simulink subsystem "quatquad_controller_sim"  (R2021b)
settings: Solver=VariableStepAuto  StartTime=0.0  StopTime=10.0  RelTol=1e-3
values from neighbouring files (symbols this model uses):
  K_d1 = K_d1_lqr    [quatquad_main.m]
  K_d2 = K_d2_lqr    [quatquad_main.m]
  K_e = K_e_lqr    [quatquad_main.m]
  K_f = K_f_lqr    [quatquad_main.m]
  linearization_method = 1    [quatquad_main.m]
  S_c = [zeros(9,1),eye(9)]    [quatquad_analysis.m]
  u_eq = [9.81;0;0;0]    [quatquad_main.m]
undefined symbols (not defined in the file or in its folder): K_alt_f, K_att_f, K_attr_f, T_e
libraries: simulink x3
settings Model: Creator=vifre  LastModifiedBy=vifre

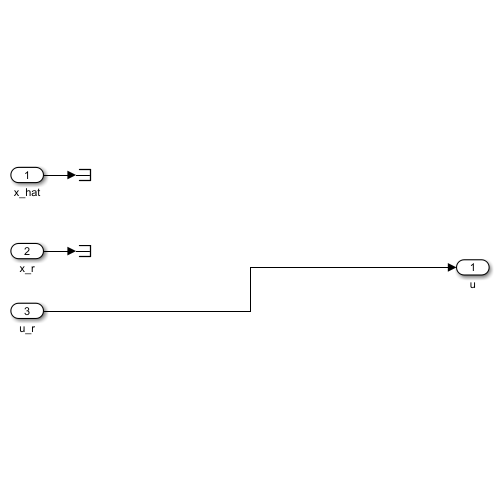
[thumbnail: Simulink's stored preview of the top-level diagram]
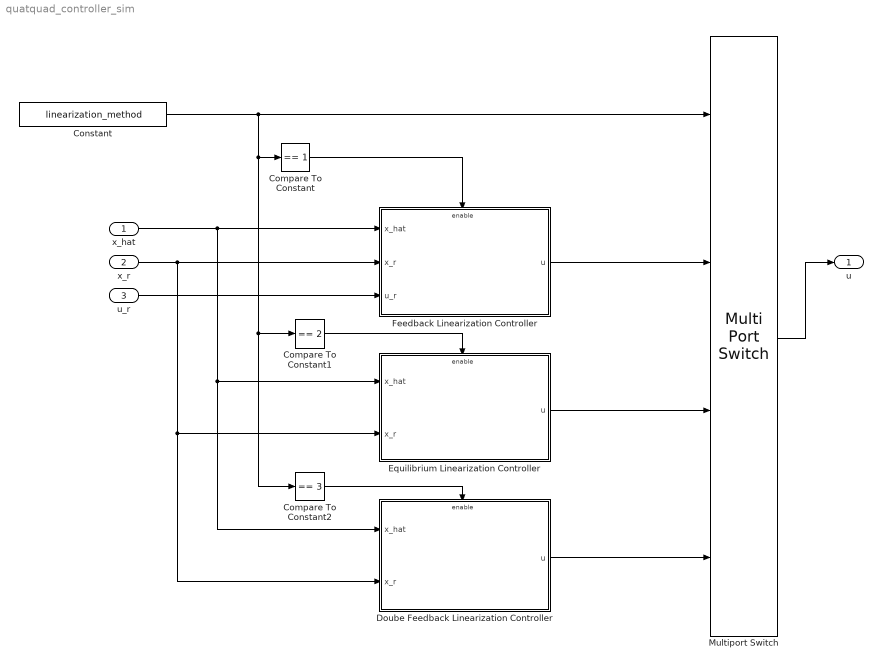
== system quatquad_controller_sim ==
  x_hat : Inport
  x_r : Inport  Port=2
  u_r : Inport  Port=3
  Compare To Constant : simulink/Logic and Bit Operations/Compare To Constant  relop===  const=1  OutDataTypeStr=boolean
  Compare To Constant1 : simulink/Logic and Bit Operations/Compare To Constant  relop===  const=2  OutDataTypeStr=boolean
  Compare To Constant2 : simulink/Logic and Bit Operations/Compare To Constant  relop===  const=3  OutDataTypeStr=boolean
  Constant : Constant  Value=linearization_method
  Doube Feedback Linearization Controller : Subsystem
  Equilibrium Linearization Controller : Subsystem
  Feedback Linearization Controller : Subsystem
  Multiport Switch : MultiPortSwitch
  u : Outport
  wires:
  x_hat/1 -> Doube Feedback Linearization Controller/1(x_hat), Equilibrium Linearization Controller/1(x_hat), Feedback Linearization Controller/1(x_hat)
  x_r/1 -> Doube Feedback Linearization Controller/2(x_r), Equilibrium Linearization Controller/2(x_r), Feedback Linearization Controller/2(x_r)
  u_r/1 -> Feedback Linearization Controller/3(u_r)
  Equilibrium Linearization Controller/1(u) -> Multiport Switch/3
  Multiport Switch/1 -> u/1
  Feedback Linearization Controller/1(u) -> Multiport Switch/2
  Constant/1 -> Compare To Constant/1, Compare To Constant1/1, Compare To Constant2/1, Multiport Switch/1
  Doube Feedback Linearization Controller/1(u) -> Multiport Switch/4
  Compare To Constant/1 -> Feedback Linearization Controller/Enable
  Compare To Constant1/1 -> Equilibrium Linearization Controller/Enable
  Compare To Constant2/1 -> Doube Feedback Linearization Controller/Enable

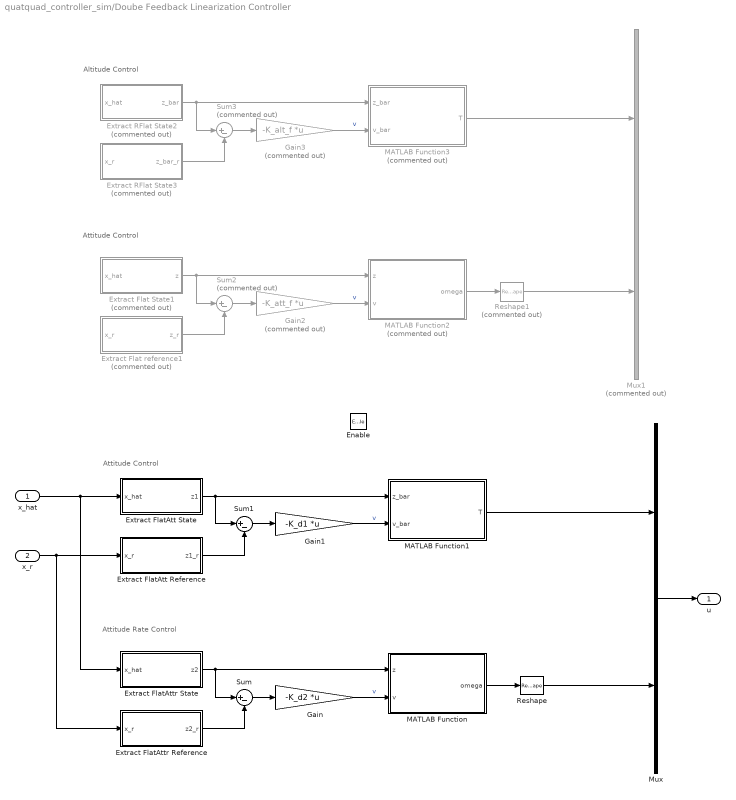
== system quatquad_controller_sim/Doube Feedback Linearization Controller ==
  note: Attitude Control
  note: Attitude Rate Control
  note: Attitude Control
  note: Altitude Control
  x_hat : Inport
  x_r : Inport  Port=2
  Enable : EnablePort
  Extract Flat State1 : Subsystem  Commented=on
  Extract Flat reference1 : Subsystem  Commented=on
  Extract FlatAtt Reference : Subsystem
  Extract FlatAtt State : Subsystem
  Extract FlatAttr Reference : Subsystem
  Extract FlatAttr State : Subsystem
  Extract RFlat State2 : Subsystem  Commented=on
  Extract RFlat State3 : Subsystem  Commented=on
  Gain : Gain  Gain=-K_d2  Multiplication=Matrix(K*u) (u vector)
  Gain1 : Gain  Gain=-K_d1  Multiplication=Matrix(K*u) (u vector)
  Gain2 : Gain  Commented=on  Gain=-K_att_f  Multiplication=Matrix(K*u) (u vector)
  Gain3 : Gain  Commented=on  Gain=-K_alt_f  Multiplication=Matrix(K*u) (u vector)
  MATLAB Function : MATLAB Function  TreatAsAtomicUnit=on
  MATLAB Function1 : MATLAB Function  TreatAsAtomicUnit=on
  MATLAB Function2 : MATLAB Function  Commented=on  TreatAsAtomicUnit=on
  MATLAB Function3 : MATLAB Function  Commented=on  TreatAsAtomicUnit=on
  Mux : Mux  Inputs=2
  Mux1 : Mux  Commented=on  Inputs=2
  Reshape : Reshape
  Reshape1 : Reshape  Commented=on
  Sum : Sum  Inputs=|+-
  Sum1 : Sum  Inputs=|+-
  Sum2 : Sum  Commented=on  Inputs=|+-
  Sum3 : Sum  Commented=on  Inputs=|+-
  u : Outport
  wires:
  x_r/1 -> Extract FlatAtt Reference/1(x_r), Extract FlatAttr Reference/1(x_r)
  x_hat/1 -> Extract FlatAtt State/1(x_hat), Extract FlatAttr State/1(x_hat)
  Mux/1 -> u/1
  Extract FlatAttr State/1(z2) -> Sum/1, MATLAB Function/1(z)
  Gain/1 -> MATLAB Function/2(v)  "v"
  MATLAB Function/1(omega) -> Reshape/1
  Extract FlatAttr Reference/1(z2_r) -> Sum/2
  Sum/1 -> Gain/1
  Sum1/1 -> Gain1/1
  Extract FlatAtt Reference/1(z1_r) -> Sum1/2
  Gain1/1 -> MATLAB Function1/2(v_bar)  "v"
  Extract FlatAtt State/1(z1) -> Sum1/1, MATLAB Function1/1(z_bar)
  Reshape/1 -> Mux/2
  MATLAB Function1/1(T) -> Mux/1
  Gain3/1 -> MATLAB Function3/2(v_bar)  "v"
  Sum3/1 -> Gain3/1
  Reshape1/1 -> Mux1/2
  MATLAB Function3/1(T) -> Mux1/1
  Extract Flat State1/1(z) -> Sum2/1, MATLAB Function2/1(z)
  Sum2/1 -> Gain2/1
  Extract Flat reference1/1(z_r) -> Sum2/2
  Extract RFlat State3/1(z_bar_r) -> Sum3/2
  Extract RFlat State2/1(z_bar) -> Sum3/1, MATLAB Function3/1(z_bar)
  MATLAB Function2/1(omega) -> Reshape1/1
  Gain2/1 -> MATLAB Function2/2(v)  "v"

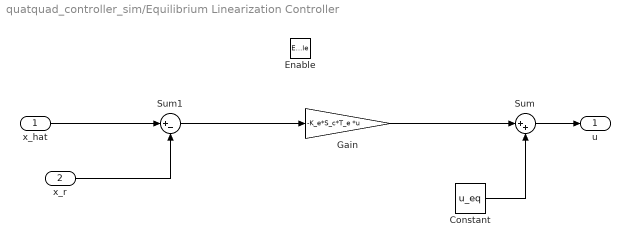
== system quatquad_controller_sim/Equilibrium Linearization Controller ==
  x_hat : Inport
  x_r : Inport  Port=2
  Enable : EnablePort
  Constant : Constant  Value=u_eq
  Gain : Gain  Gain=-K_e*S_c*T_e  Multiplication=Matrix(K*u) (u vector)
  Sum : Sum  Inputs=|++
  Sum1 : Sum  Inputs=|+-
  u : Outport
  wires:
  x_r/1 -> Sum1/2
  x_hat/1 -> Sum1/1
  Sum1/1 -> Gain/1
  Gain/1 -> Sum/1
  Constant/1 -> Sum/2
  Sum/1 -> u/1

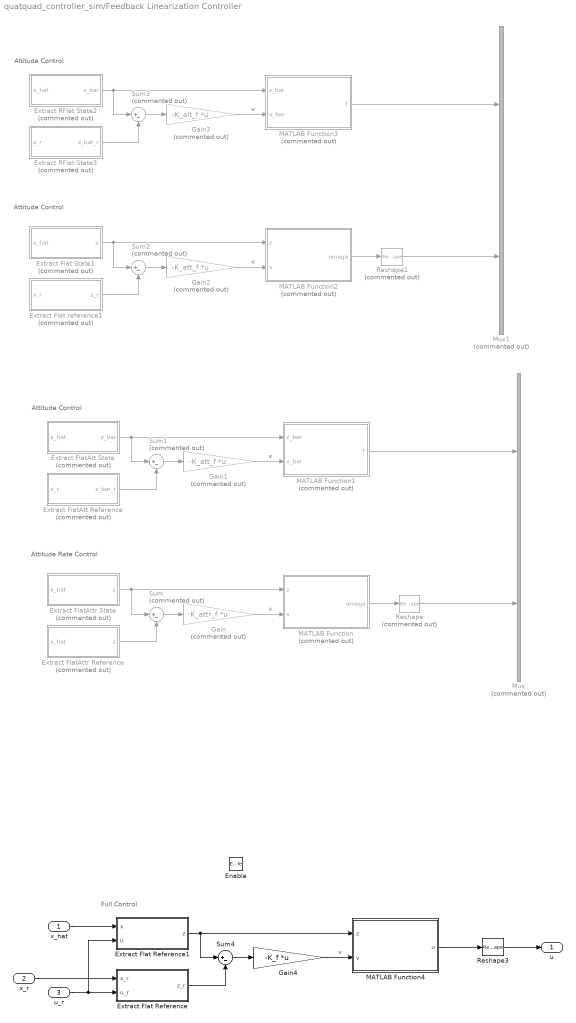
== system quatquad_controller_sim/Feedback Linearization Controller ==
  note: Full Control
  note: Altitude Control
  note: Attitude Control
  note: Attitude Rate Control
  note: Attitude Control
  x_hat : Inport
  x_r : Inport  Port=2
  u_r : Inport  Port=3
  Enable : EnablePort
  Extract Flat Reference : Subsystem
  Extract Flat Reference1 : Subsystem
  Extract Flat State1 : Subsystem  Commented=on
  Extract Flat reference1 : Subsystem  Commented=on
  Extract FlatAtt Reference : Subsystem  Commented=on
  Extract FlatAtt State : Subsystem  Commented=on
  Extract FlatAttr Reference : Subsystem  Commented=on
  Extract FlatAttr State : Subsystem  Commented=on
  Extract RFlat State2 : Subsystem  Commented=on
  Extract RFlat State3 : Subsystem  Commented=on
  Gain : Gain  Commented=on  Gain=-K_attr_f  Multiplication=Matrix(K*u) (u vector)
  Gain1 : Gain  Commented=on  Gain=-K_att_f  Multiplication=Matrix(K*u) (u vector)
  Gain2 : Gain  Commented=on  Gain=-K_att_f  Multiplication=Matrix(K*u) (u vector)
  Gain3 : Gain  Commented=on  Gain=-K_alt_f  Multiplication=Matrix(K*u) (u vector)
  Gain4 : Gain  Gain=-K_f  Multiplication=Matrix(K*u) (u vector)
  MATLAB Function : MATLAB Function  Commented=on  TreatAsAtomicUnit=on
  MATLAB Function1 : MATLAB Function  Commented=on  TreatAsAtomicUnit=on
  MATLAB Function2 : MATLAB Function  Commented=on  TreatAsAtomicUnit=on
  MATLAB Function3 : MATLAB Function  Commented=on  TreatAsAtomicUnit=on
  MATLAB Function4 : MATLAB Function  TreatAsAtomicUnit=on
  Mux : Mux  Commented=on  Inputs=2
  Mux1 : Mux  Commented=on  Inputs=2
  Reshape : Reshape  Commented=on
  Reshape1 : Reshape  Commented=on
  Reshape3 : Reshape
  Sum{,1..3} (4 alike) : Sum  Commented=on  Inputs=|+-
  Sum4 : Sum  Inputs=|+-
  u : Outport
  wires:
  u_r/1 -> Extract Flat Reference/2(u_r), Extract Flat Reference1/2(u)
  MATLAB Function4/1(u) -> Reshape3/1
  Extract Flat Reference1/1(z) -> MATLAB Function4/1(z), Sum4/1
  Extract Flat Reference/1(z_r) -> Sum4/2
  Gain4/1 -> MATLAB Function4/2(v)  "v"
  Sum4/1 -> Gain4/1
  x_r/1 -> Extract Flat Reference/1(x_r)
  x_hat/1 -> Extract Flat Reference1/1(x)
  Reshape3/1 -> u/1
  Gain2/1 -> MATLAB Function2/2(v)  "v"
  MATLAB Function2/1(omega) -> Reshape1/1
  Extract RFlat State2/1(z_bar) -> MATLAB Function3/1(z_bar), Sum3/1
  Extract RFlat State3/1(z_bar_r) -> Sum3/2
  Extract Flat reference1/1(z_r) -> Sum2/2
  Sum2/1 -> Gain2/1
  Extract Flat State1/1(z) -> MATLAB Function2/1(z), Sum2/1
  MATLAB Function3/1(T) -> Mux1/1
  Reshape1/1 -> Mux1/2
  Sum3/1 -> Gain3/1
  Gain3/1 -> MATLAB Function3/2(v_bar)  "v"
  MATLAB Function1/1(T) -> Mux/1
  Reshape/1 -> Mux/2
  Extract FlatAtt State/1(z_bar) -> MATLAB Function1/1(z_bar), Sum1/1
  Gain1/1 -> MATLAB Function1/2(v_bar)  "v"
  Extract FlatAtt Reference/1(z_bar_r) -> Sum1/2
  Sum1/1 -> Gain1/1
  Sum/1 -> Gain/1
  Extract FlatAttr Reference/1(z) -> Sum/2
  MATLAB Function/1(omega) -> Reshape/1
  Gain/1 -> MATLAB Function/2(v)  "v"
  Extract FlatAttr State/1(z) -> MATLAB Function/1(z), Sum/1

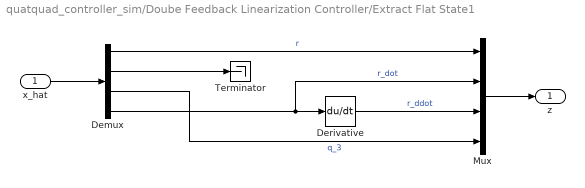
== system quatquad_controller_sim/Doube Feedback Linearization Controller/Extract Flat State1 ==
  x_hat : Inport
  Demux : Demux  Outputs=[3 3 1 3]
  Derivative : Derivative
  Mux : Mux
  Terminator : Terminator
  z : Outport
  wires:
  x_hat/1 -> Demux/1
  Demux/1 -> Mux/1  "r"
  Derivative/1 -> Mux/3  "r_ddot"
  Mux/1 -> z/1
  Demux/3 -> Mux/4  "q_3"
  Demux/2 -> Terminator/1
  Demux/4 -> Mux/2, Derivative/1  "r_dot"

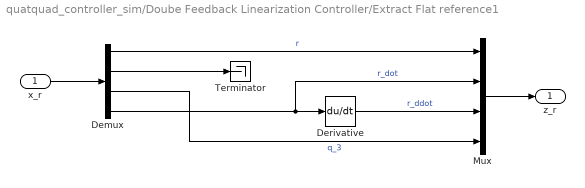
== system quatquad_controller_sim/Doube Feedback Linearization Controller/Extract Flat reference1 ==
  x_r : Inport
  Demux : Demux  Outputs=[3 3 1 3]
  Derivative : Derivative
  Mux : Mux
  Terminator : Terminator
  z_r : Outport
  wires:
  Demux/4 -> Derivative/1, Mux/2  "r_dot"
  Demux/2 -> Terminator/1
  Demux/3 -> Mux/4  "q_3"
  Mux/1 -> z_r/1
  Derivative/1 -> Mux/3  "r_ddot"
  Demux/1 -> Mux/1  "r"
  x_r/1 -> Demux/1

== system quatquad_controller_sim/Doube Feedback Linearization Controller/Extract FlatAtt Reference ==
  x_r : Inport
  Demux : Demux  Outputs=[3 4 3]
  Mux : Mux  Inputs=2
  Terminator : Terminator
  z1_r : Outport
  wires:
  Demux/3 -> Mux/2  "r_dot"
  x_r/1 -> Demux/1
  Demux/1 -> Mux/1  "r"
  Mux/1 -> z1_r/1
  Demux/2 -> Terminator/1

== system quatquad_controller_sim/Doube Feedback Linearization Controller/Extract FlatAtt State ==
  x_hat : Inport
  Demux : Demux  Outputs=[3 4 3]
  Mux : Mux  Inputs=2
  Terminator : Terminator
  z1 : Outport
  wires:
  Demux/2 -> Terminator/1
  Mux/1 -> z1/1
  Demux/1 -> Mux/1  "r"
  x_hat/1 -> Demux/1
  Demux/3 -> Mux/2  "r_dot"

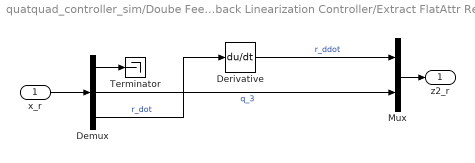
== system quatquad_controller_sim/Doube Feedback Linearization Controller/Extract FlatAttr Reference ==
  x_r : Inport
  Demux : Demux  Outputs=[6 1 3]
  Derivative : Derivative
  Mux : Mux  Inputs=2
  Terminator : Terminator
  z2_r : Outport
  wires:
  x_r/1 -> Demux/1
  Derivative/1 -> Mux/1  "r_ddot"
  Mux/1 -> z2_r/1
  Demux/1 -> Terminator/1
  Demux/2 -> Mux/2  "q_3"
  Demux/3 -> Derivative/1  "r_dot"

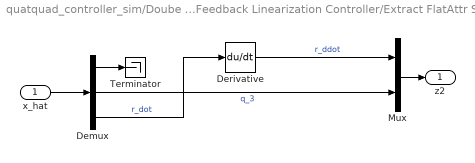
== system quatquad_controller_sim/Doube Feedback Linearization Controller/Extract FlatAttr State ==
  x_hat : Inport
  Demux : Demux  Outputs=[6 1 3]
  Derivative : Derivative
  Mux : Mux  Inputs=2
  Terminator : Terminator
  z2 : Outport
  wires:
  x_hat/1 -> Demux/1
  Derivative/1 -> Mux/1  "r_ddot"
  Mux/1 -> z2/1
  Demux/1 -> Terminator/1
  Demux/2 -> Mux/2  "q_3"
  Demux/3 -> Derivative/1  "r_dot"

== system quatquad_controller_sim/Doube Feedback Linearization Controller/Extract RFlat State2 ==
  x_hat : Inport
  Demux : Demux  Outputs=[3 4 3]
  Mux : Mux  Inputs=2
  Terminator : Terminator
  z_bar : Outport
  wires:
  Demux/2 -> Terminator/1
  Mux/1 -> z_bar/1
  Demux/1 -> Mux/1  "r"
  x_hat/1 -> Demux/1
  Demux/3 -> Mux/2  "r_dot"

== system quatquad_controller_sim/Doube Feedback Linearization Controller/Extract RFlat State3 ==
  x_r : Inport
  Demux : Demux  Outputs=[3 4 3]
  Mux : Mux  Inputs=2
  Terminator : Terminator
  z_bar_r : Outport
  wires:
  Demux/3 -> Mux/2  "r_dot"
  x_r/1 -> Demux/1
  Demux/1 -> Mux/1  "r"
  Mux/1 -> z_bar_r/1
  Demux/2 -> Terminator/1

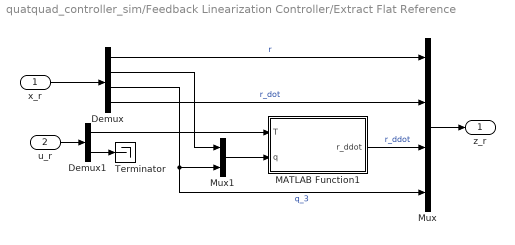
== system quatquad_controller_sim/Feedback Linearization Controller/Extract Flat Reference ==
  x_r : Inport
  u_r : Inport  Port=2
  Demux : Demux  Outputs=[3 3 1 3]
  Demux1 : Demux  Outputs=[1 3]
  MATLAB Function1 : MATLAB Function  TreatAsAtomicUnit=on
  Mux : Mux
  Mux1 : Mux  Inputs=2
  Terminator : Terminator
  z_r : Outport
  wires:
  u_r/1 -> Demux1/1
  Demux1/1 -> MATLAB Function1/1(T)
  Demux1/2 -> Terminator/1
  Mux1/1 -> MATLAB Function1/2(q)
  MATLAB Function1/1(r_ddot) -> Mux/3  "r_ddot"
  Demux/2 -> Mux1/1
  Mux/1 -> z_r/1
  Demux/1 -> Mux/1  "r"
  x_r/1 -> Demux/1
  Demux/4 -> Mux/2  "r_dot"
  Demux/3 -> Mux/4, Mux1/2  "q_3"

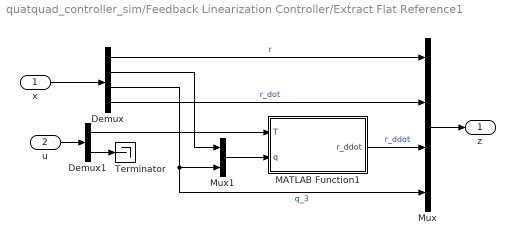
== system quatquad_controller_sim/Feedback Linearization Controller/Extract Flat Reference1 ==
  x : Inport
  u : Inport  Port=2
  Demux : Demux  Outputs=[3 3 1 3]
  Demux1 : Demux  Outputs=[1 3]
  MATLAB Function1 : MATLAB Function  TreatAsAtomicUnit=on
  Mux : Mux
  Mux1 : Mux  Inputs=2
  Terminator : Terminator
  z : Outport
  wires:
  Demux/3 -> Mux1/2, Mux/4  "q_3"
  Demux/4 -> Mux/2  "r_dot"
  x/1 -> Demux/1
  Demux/1 -> Mux/1  "r"
  Mux/1 -> z/1
  Demux/2 -> Mux1/1
  MATLAB Function1/1(r_ddot) -> Mux/3  "r_ddot"
  Mux1/1 -> MATLAB Function1/2(q)
  Demux1/2 -> Terminator/1
  Demux1/1 -> MATLAB Function1/1(T)
  u/1 -> Demux1/1

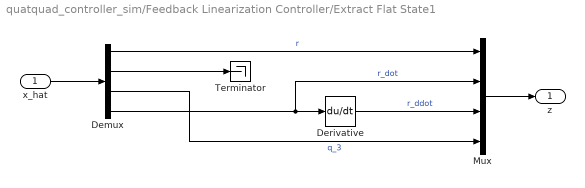
== system quatquad_controller_sim/Feedback Linearization Controller/Extract Flat State1 ==
  x_hat : Inport
  Demux : Demux  Outputs=[3 3 1 3]
  Derivative : Derivative
  Mux : Mux
  Terminator : Terminator
  z : Outport
  wires:
  Demux/4 -> Derivative/1, Mux/2  "r_dot"
  Demux/2 -> Terminator/1
  Demux/3 -> Mux/4  "q_3"
  Mux/1 -> z/1
  Derivative/1 -> Mux/3  "r_ddot"
  Demux/1 -> Mux/1  "r"
  x_hat/1 -> Demux/1

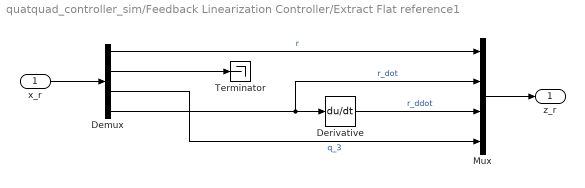
== system quatquad_controller_sim/Feedback Linearization Controller/Extract Flat reference1 ==
  x_r : Inport
  Demux : Demux  Outputs=[3 3 1 3]
  Derivative : Derivative
  Mux : Mux
  Terminator : Terminator
  z_r : Outport
  wires:
  x_r/1 -> Demux/1
  Demux/1 -> Mux/1  "r"
  Derivative/1 -> Mux/3  "r_ddot"
  Mux/1 -> z_r/1
  Demux/3 -> Mux/4  "q_3"
  Demux/2 -> Terminator/1
  Demux/4 -> Mux/2, Derivative/1  "r_dot"

== system quatquad_controller_sim/Feedback Linearization Controller/Extract FlatAtt Reference ==
  x_r : Inport
  Demux : Demux  Outputs=[3 4 3]
  Mux : Mux  Inputs=2
  Terminator : Terminator
  z_bar_r : Outport
  wires:
  Demux/2 -> Terminator/1
  Mux/1 -> z_bar_r/1
  Demux/1 -> Mux/1  "r"
  x_r/1 -> Demux/1
  Demux/3 -> Mux/2  "r_dot"

== system quatquad_controller_sim/Feedback Linearization Controller/Extract FlatAtt State ==
  x_hat : Inport
  Demux : Demux  Outputs=[3 4 3]
  Mux : Mux  Inputs=2
  Terminator : Terminator
  z_bar : Outport
  wires:
  Demux/3 -> Mux/2  "r_dot"
  x_hat/1 -> Demux/1
  Demux/1 -> Mux/1  "r"
  Mux/1 -> z_bar/1
  Demux/2 -> Terminator/1

== system quatquad_controller_sim/Feedback Linearization Controller/Extract FlatAttr Reference ==
  x_hat : Inport
  Demux : Demux  Outputs=[6 1 3]
  Derivative : Derivative
  Mux : Mux  Inputs=2
  Terminator : Terminator
  z : Outport
  wires:
  Demux/3 -> Derivative/1  "r_dot"
  Demux/2 -> Mux/2  "q_3"
  Demux/1 -> Terminator/1
  Mux/1 -> z/1
  Derivative/1 -> Mux/1  "r_ddot"
  x_hat/1 -> Demux/1

== system quatquad_controller_sim/Feedback Linearization Controller/Extract FlatAttr State ==
  x_hat : Inport
  Demux : Demux  Outputs=[6 1 3]
  Derivative : Derivative
  Mux : Mux  Inputs=2
  Terminator : Terminator
  z : Outport
  wires:
  Demux/3 -> Derivative/1  "r_dot"
  Demux/2 -> Mux/2  "q_3"
  Demux/1 -> Terminator/1
  Mux/1 -> z/1
  Derivative/1 -> Mux/1  "r_ddot"
  x_hat/1 -> Demux/1

== system quatquad_controller_sim/Feedback Linearization Controller/Extract RFlat State2 ==
  x_hat : Inport
  Demux : Demux  Outputs=[3 4 3]
  Mux : Mux  Inputs=2
  Terminator : Terminator
  z_bar : Outport
  wires:
  Demux/3 -> Mux/2  "r_dot"
  x_hat/1 -> Demux/1
  Demux/1 -> Mux/1  "r"
  Mux/1 -> z_bar/1
  Demux/2 -> Terminator/1

== system quatquad_controller_sim/Feedback Linearization Controller/Extract RFlat State3 ==
  x_r : Inport
  Demux : Demux  Outputs=[3 4 3]
  Mux : Mux  Inputs=2
  Terminator : Terminator
  z_bar_r : Outport
  wires:
  Demux/2 -> Terminator/1
  Mux/1 -> z_bar_r/1
  Demux/1 -> Mux/1  "r"
  x_r/1 -> Demux/1
  Demux/3 -> Mux/2  "r_dot"

== matlab function quatquad_controller_sim/Feedback Linearization Controller/MATLAB Function1 ==
  data: z_bar input; T output; v_bar input
function T = recover_att(z_bar, v_bar)
g = 9.81;
z_W = [0;0;1];
T = norm(v_bar + g*z_W);

== matlab function quatquad_controller_sim/Feedback Linearization Controller/MATLAB Function2 ==
  data: z input; omega output; v input
function omega = recover_att(z, v)
g = 9.81;
u = zeros(4,1);
r = z(1:3);
r_dot = z(4:6);
r_ddot = z(7:9);
q_3 = z(10);
r_dddot = v(1:3);
q_dot_3 = v(4);
z_W = [0;0;1];
T = norm(r_ddot+g*z_W);
q_0 = sqrt((r_ddot(3)+g)/T-q_3^2+1/2);
q_1 = (q_3*r_ddot(1) - q_0*r_ddot(2))/(2*T*(q_0^2+q_3^2));
q_2 = (q_0*r_ddot(1) + q_3*r_ddot(2))/(2*T*(q_0^2+q_3^2));
q = [q_0;q_1;q_2;q_3];
z_B = [2*(q(1)*q(3) + q(2)*q(4));
       -2*(q(1)*q(2) - q(3)*q(4));
       (q(1)^2 - q(2)^2 - q(3)^2 + q(4)^2)];
T_dot = dot(r_dddot,z_B);
q_dot_0 = 1/(2*q_0)*((T*r_dddot(3)-T_dot)/(2*T^2) - 2*q_3*q_dot_3);
num_q1 = q_3*r_ddot(1) - q_0*r_ddot(2);
num_q2 = q_0*r_ddot(1) + q_3*r_ddot(2);
num_q1_dot = q_dot_3*r_ddot(1) + q_3*r_dddot(1) - q_dot_0*r_ddot(2) - q_0*r_dddot(2);
num_q2_dot = q_dot_0*r_ddot(1) + q_0*r_dddot(1) + q_dot_3*r_ddot(2) + q_3*r_dddot(2); 
den = (2*T*(q_0^2 + q_3^2))^-1;
den_dot = -(2*T*(q_0^2+q_3^2))^(-2)*(2*T_dot*(q_0^2+q_3^2) + 2*T*(2*q_0*q_dot_0 + 2*q_3*q_dot_3));
q_dot_1 = num_q1_dot*den + den_dot*num_q1;
q_dot_2 = num_q2_dot*den + den_dot*num_q2;
% q_dot = [q_dot_0;q_dot_1;q_dot_2;q_dot_3];
omega = 2*[q_0*q_dot_1 - q_1*q_dot_0 - q_2*q_dot_3 + q_3*q_dot_2;
           q_0*q_dot_2 - q_2*q_dot_0 + q_1*q_dot_3 - q_3*q_dot_1;
           q_0*q_dot_3 - q_1*q_dot_2 + q_2*q_dot_1 - q_3*q_dot_0];
% u(1) = T;
% u(2:4) = omega;

== matlab function quatquad_controller_sim/Feedback Linearization Controller/MATLAB Function3 ==
  data: z_bar input; T output; v_bar input
function T = recover_alt(z_bar, v_bar)
g = 9.81;
z_W = [0;0;1];
T = norm(v_bar + g*z_W);

== matlab function quatquad_controller_sim/Feedback Linearization Controller/MATLAB Function4 ==
  data: z input; u output; v input
function u = recover(z, v)
g = 9.81;
z_W = [0;0;1];
g = 9.81;
r_ddot = v(1:3);
q_3 = z(10);
r_dddot = v(4:6);
q_dot_3 = v(7);
T = norm(r_ddot+g*z_W);
q_0 = sqrt((r_ddot(3)+g)/(2*T)-q_3^2+1/2);
q_1 = (q_3*r_ddot(1) - q_0*r_ddot(2))/(2*T*(q_0^2+q_3^2));
q_2 = (q_0*r_ddot(1) + q_3*r_ddot(2))/(2*T*(q_0^2+q_3^2));
q = [q_0;q_1;q_2;q_3];
z_B = [2*(q(1)*q(3) + q(2)*q(4));
       -2*(q(1)*q(2) - q(3)*q(4));
       (q(1)^2 - q(2)^2 - q(3)^2 + q(4)^2)];
T_dot = dot(r_dddot,z_B);
q_dot_0 = 1/(2*q_0)*((T*r_dddot(3)-T_dot)/(2*T^2) - 2*q_3*q_dot_3);
num_q1 = q_3*r_ddot(1) - q_0*r_ddot(2);
num_q2 = q_0*r_ddot(1) + q_3*r_ddot(2);
num_q1_dot = q_dot_3*r_ddot(1) + q_3*r_dddot(1) - q_dot_0*r_ddot(2) - q_0*r_dddot(2);
num_q2_dot = q_dot_0*r_ddot(1) + q_0*r_dddot(1) + q_dot_3*r_ddot(2) + q_3*r_dddot(2); 
den = (2*T*(q_0^2 + q_3^2))^-1;
den_dot = -(2*T*(q_0^2+q_3^2))^(-2)*(2*T_dot*(q_0^2+q_3^2) + 2*T*(2*q_0*q_dot_0 + 2*q_3*q_dot_3));
q_dot_1 = num_q1_dot*den + den_dot*num_q1;
q_dot_2 = num_q2_dot*den + den_dot*num_q2;
omega = 2*[q_0*q_dot_1 - q_1*q_dot_0 - q_2*q_dot_3 + q_3*q_dot_2;
           q_0*q_dot_2 - q_2*q_dot_0 + q_1*q_dot_3 - q_3*q_dot_1;
           q_0*q_dot_3 - q_1*q_dot_2 + q_2*q_dot_1 - q_3*q_dot_0];
u = [T; omega];

== matlab function quatquad_controller_sim/Feedback Linearization Controller/Extract Flat Reference1/MATLAB Function1 ==
  data: T input; r_ddot output; q input
function r_ddot = Newton(T,q)
x_ddot = 2*T*(q(1)*q(3) + q(2)*q(4));
y_ddot = -2*T*(q(1)*q(2) - q(3)*q(4));
z_ddot = T*(q(1)^2 - q(2)^2 - q(3)^2 + q(4)^2) - 9.81;
r_ddot = [x_ddot;y_ddot;z_ddot];
end

== matlab function quatquad_controller_sim/Feedback Linearization Controller/Extract Flat Reference/MATLAB Function1 ==
  data: T input; r_ddot output; q input
function r_ddot = Newton(T,q)
x_ddot = 2*T*(q(1)*q(3) + q(2)*q(4));
y_ddot = -2*T*(q(1)*q(2) - q(3)*q(4));
z_ddot = T*(q(1)^2 - q(2)^2 - q(3)^2 + q(4)^2) - 9.81;
r_ddot = [x_ddot;y_ddot;z_ddot];
end

== matlab function quatquad_controller_sim/Doube Feedback Linearization Controller/MATLAB Function ==
  data: z input; omega output; v input
function omega = recover_attr(z, v)
g = 9.81;
r_ddot = z(1:3);
q_3 = z(4);
r_dddot = v(1:3);
q_dot_3 = v(4);
z_W = [0;0;1];
T = norm(r_ddot+g*z_W);
q_0 = sqrt((r_ddot(3)+g)/(2*T)-q_3^2+1/2);
q_1 = (q_3*r_ddot(1) - q_0*r_ddot(2))/(2*T*(q_0^2+q_3^2));
q_2 = (q_0*r_ddot(1) + q_3*r_ddot(2))/(2*T*(q_0^2+q_3^2));
q = [q_0;q_1;q_2;q_3];
z_B = [2*(q(1)*q(3) + q(2)*q(4));
       -2*(q(1)*q(2) - q(3)*q(4));
       (q(1)^2 - q(2)^2 - q(3)^2 + q(4)^2)];
T_dot = dot(r_dddot,z_B);
q_dot_0 = 1/(2*q_0)*((T*r_dddot(3)-T_dot)/(2*T^2) - 2*q_3*q_dot_3);
num_q1 = q_3*r_ddot(1) - q_0*r_ddot(2);
num_q2 = q_0*r_ddot(1) + q_3*r_ddot(2);
num_q1_dot = q_dot_3*r_ddot(1) + q_3*r_dddot(1) - q_dot_0*r_ddot(2) - q_0*r_dddot(2);
num_q2_dot = q_dot_0*r_ddot(1) + q_0*r_dddot(1) + q_dot_3*r_ddot(2) + q_3*r_dddot(2); 
den = (2*T*(q_0^2 + q_3^2))^-1;
den_dot = -(2*T*(q_0^2+q_3^2))^(-2)*(2*T_dot*(q_0^2+q_3^2) + 2*T*(2*q_0*q_dot_0 + 2*q_3*q_dot_3));
q_dot_1 = num_q1_dot*den + den_dot*num_q1;
q_dot_2 = num_q2_dot*den + den_dot*num_q2;
omega = 2*[q_0*q_dot_1 - q_1*q_dot_0 - q_2*q_dot_3 + q_3*q_dot_2;
           q_0*q_dot_2 - q_2*q_dot_0 + q_1*q_dot_3 - q_3*q_dot_1;
           q_0*q_dot_3 - q_1*q_dot_2 + q_2*q_dot_1 - q_3*q_dot_0];

== matlab function quatquad_controller_sim/Doube Feedback Linearization Controller/MATLAB Function1 ==
  data: z_bar input; T output; v_bar input
function T = recover_att(z_bar, v_bar)
g = 9.81;
z_W = [0;0;1];
T = norm(v_bar + g*z_W);

== matlab function quatquad_controller_sim/Feedback Linearization Controller/MATLAB Function ==
  data: z input; omega output; v input
function omega = recover_attr(z, v)
g = 9.81;
r_ddot = z(1:3);
q_3 = z(4);
r_dddot = v(1:3);
q_dot_3 = v(4);
z_W = [0;0;1];
T = norm(r_ddot+g*z_W);
q_0 = sqrt((r_ddot(3)+g)/T-q_3^2+1/2);
q_1 = (q_3*r_ddot(1) - q_0*r_ddot(2))/(2*T*(q_0^2+q_3^2));
q_2 = (q_0*r_ddot(1) + q_3*r_ddot(2))/(2*T*(q_0^2+q_3^2));
q = [q_0;q_1;q_2;q_3];
z_B = [2*(q(1)*q(3) + q(2)*q(4));
       -2*(q(1)*q(2) - q(3)*q(4));
       (q(1)^2 - q(2)^2 - q(3)^2 + q(4)^2)];
T_dot = dot(r_dddot,z_B);
q_dot_0 = 1/(2*q_0)*((T*r_dddot(3)-T_dot)/(2*T^2) - 2*q_3*q_dot_3);
num_q1 = q_3*r_ddot(1) - q_0*r_ddot(2);
num_q2 = q_0*r_ddot(1) + q_3*r_ddot(2);
num_q1_dot = q_dot_3*r_ddot(1) + q_3*r_dddot(1) - q_dot_0*r_ddot(2) - q_0*r_dddot(2);
num_q2_dot = q_dot_0*r_ddot(1) + q_0*r_dddot(1) + q_dot_3*r_ddot(2) + q_3*r_dddot(2); 
den = (2*T*(q_0^2 + q_3^2))^-1;
den_dot = -(2*T*(q_0^2+q_3^2))^(-2)*(2*T_dot*(q_0^2+q_3^2) + 2*T*(2*q_0*q_dot_0 + 2*q_3*q_dot_3));
q_dot_1 = num_q1_dot*den + den_dot*num_q1;
q_dot_2 = num_q2_dot*den + den_dot*num_q2;
omega = 2*[q_0*q_dot_1 - q_1*q_dot_0 - q_2*q_dot_3 + q_3*q_dot_2;
           q_0*q_dot_2 - q_2*q_dot_0 + q_1*q_dot_3 - q_3*q_dot_1;
           q_0*q_dot_3 - q_1*q_dot_2 + q_2*q_dot_1 - q_3*q_dot_0];

== matlab function quatquad_controller_sim/Doube Feedback Linearization Controller/MATLAB Function2 ==
  data: z input; omega output; v input
function omega = recover_att(z, v)
g = 9.81;
u = zeros(4,1);
r = z(1:3);
r_dot = z(4:6);
r_ddot = z(7:9);
q_3 = z(10);
r_dddot = v(1:3);
q_dot_3 = v(4);
z_W = [0;0;1];
T = norm(r_ddot+g*z_W);
q_0 = sqrt((r_ddot(3)+g)/T-q_3^2+1/2);
q_1 = (q_3*r_ddot(1) - q_0*r_ddot(2))/(2*T*(q_0^2+q_3^2));
q_2 = (q_0*r_ddot(1) + q_3*r_ddot(2))/(2*T*(q_0^2+q_3^2));
q = [q_0;q_1;q_2;q_3];
z_B = [2*(q(1)*q(3) + q(2)*q(4));
       -2*(q(1)*q(2) - q(3)*q(4));
       (q(1)^2 - q(2)^2 - q(3)^2 + q(4)^2)];
T_dot = dot(r_dddot,z_B);
q_dot_0 = 1/(2*q_0)*((T*r_dddot(3)-T_dot)/(2*T^2) - 2*q_3*q_dot_3);
num_q1 = q_3*r_ddot(1) - q_0*r_ddot(2);
num_q2 = q_0*r_ddot(1) + q_3*r_ddot(2);
num_q1_dot = q_dot_3*r_ddot(1) + q_3*r_dddot(1) - q_dot_0*r_ddot(2) - q_0*r_dddot(2);
num_q2_dot = q_dot_0*r_ddot(1) + q_0*r_dddot(1) + q_dot_3*r_ddot(2) + q_3*r_dddot(2); 
den = (2*T*(q_0^2 + q_3^2))^-1;
den_dot = -(2*T*(q_0^2+q_3^2))^(-2)*(2*T_dot*(q_0^2+q_3^2) + 2*T*(2*q_0*q_dot_0 + 2*q_3*q_dot_3));
q_dot_1 = num_q1_dot*den + den_dot*num_q1;
q_dot_2 = num_q2_dot*den + den_dot*num_q2;
% q_dot = [q_dot_0;q_dot_1;q_dot_2;q_dot_3];
omega = 2*[q_0*q_dot_1 - q_1*q_dot_0 - q_2*q_dot_3 + q_3*q_dot_2;
           q_0*q_dot_2 - q_2*q_dot_0 + q_1*q_dot_3 - q_3*q_dot_1;
           q_0*q_dot_3 - q_1*q_dot_2 + q_2*q_dot_1 - q_3*q_dot_0];
% u(1) = T;
% u(2:4) = omega;

== matlab function quatquad_controller_sim/Doube Feedback Linearization Controller/MATLAB Function3 ==
  data: z_bar input; T output; v_bar input
function T = recover_alt(z_bar, v_bar)
g = 9.81;
z_W = [0;0;1];
T = norm(v_bar + g*z_W);
